simulink model "sim_Start_2021b"  (R2022a)
settings: Solver=FixedStepDiscrete  StartTime=0.0  StopTime=30  FixedStep=0.01  RelTol=1e-3
undefined symbols (not defined in the file): InputPWM, WheelSpeed
libraries: mobileRoboticsTrainingLib x6, simulink x2
settings Model: Creator=Boitumelo  LastModifiedBy=Admin
settings DebuggingCC: UnconnectedInputMsg=warning  UnconnectedOutputMsg=warning  UnconnectedLineMsg=warning
settings RTWCC: DLArmComputeVersion=19.05

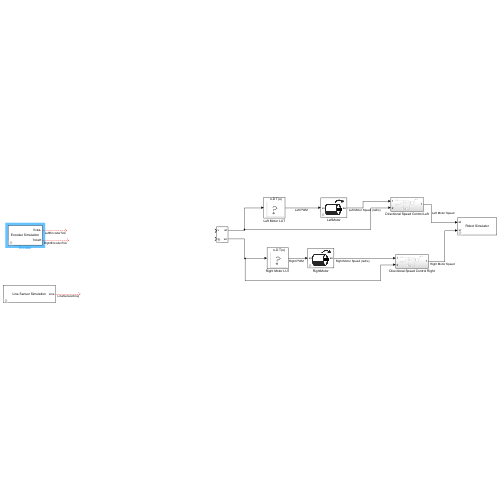
[thumbnail: Simulink's stored preview of the top-level diagram]
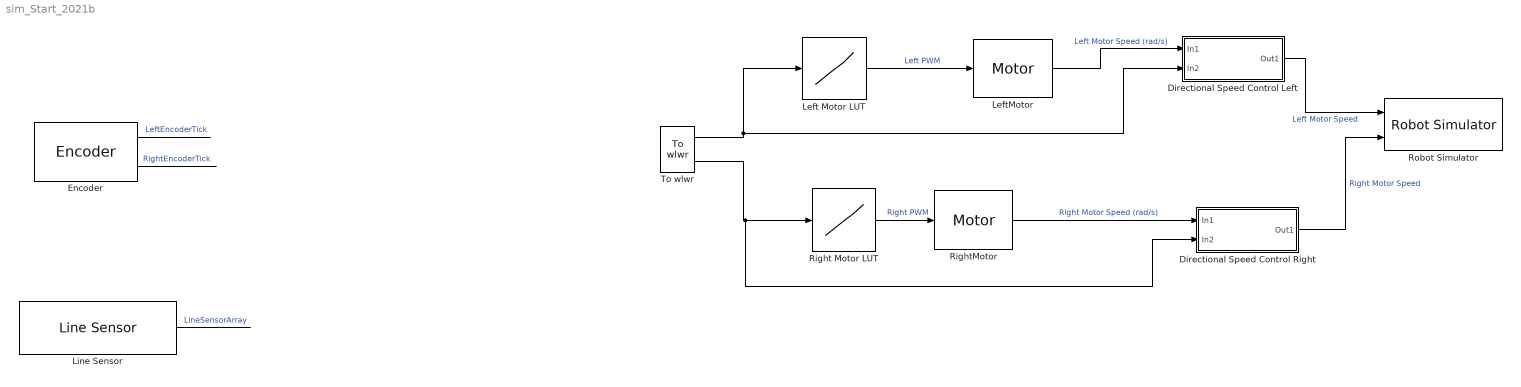
== system sim_Start_2021b ==
  Directional Speed Control Left : Subsystem
  Directional Speed Control Right : Subsystem
  Encoder : mobileRoboticsTrainingLib/Encoder  axleLength=axleLength  wheelR=wheelR  ticksPerRot=ticksPerRot
      settings: SourceProductName=Mobile Robotics Training Library
  Left Motor LUT : Lookup_n-D  NumberOfTableDimensions=1  BreakpointsForDimension1=WheelSpeed  Table=InputPWM  InterpMethod=Nearest  ExtrapMethod=Clip  InternalRulePriority=Speed  RndMeth=Simplest
  LeftMotor : mobileRoboticsTrainingLib/Motor  motorPlant=wheelMotorModel  sensorType=Speed
      settings: SourceProductName=Mobile Robotics Training Library
  Line Sensor : mobileRoboticsTrainingLib/Line Sensor  mapVariable=mapForSim  envVal=1  lineVal=0  sensOff=[0 0; 0 0; 0 0; 0 0]
      settings: SourceProductName=Mobile Robotics Training Library
  Right Motor LUT : Lookup_n-D  NumberOfTableDimensions=1  BreakpointsForDimension1=WheelSpeed  Table=InputPWM  InterpMethod=Nearest  ExtrapMethod=Clip  InternalRulePriority=Speed  RndMeth=Simplest
  RightMotor : mobileRoboticsTrainingLib/Motor  motorPlant=wheelMotorModel  sensorType=Speed
      settings: SourceProductName=Mobile Robotics Training Library
  Robot Simulator : mobileRoboticsTrainingLib/Robot Simulator  Priority=99  mapVar=mapForSim  startX=0.2126  startY=0.077048  startTheta=0  axleLength=axleLength  wheelR=wheelR
  To wlwr : mobileRoboticsTrainingLib/To wlwr  axleLength=0.1  wheelR=0.05
  wires:
  Directional Speed Control Left/1(Out1) -> Robot Simulator/1  "Left Motor Speed"
  Right Motor LUT/1 -> RightMotor/1  "Right PWM"
  Left Motor LUT/1 -> LeftMotor/1  "Left PWM"
  Encoder/1 -> ?  "LeftEncoderTick"
  Encoder/2 -> ?  "RightEncoderTick"
  To wlwr/1 -> Directional Speed Control Left/2(In2), Left Motor LUT/1
  To wlwr/2 -> Directional Speed Control Right/2(In2), Right Motor LUT/1
  Line Sensor/1 -> ?  "LineSensorArray"
  RightMotor/1 -> Directional Speed Control Right/1(In1)  "Right Motor Speed (rad/s)"
  LeftMotor/1 -> Directional Speed Control Left/1(In1)  "Left Motor Speed (rad/s)"
  Directional Speed Control Right/1(Out1) -> Robot Simulator/2  "Right Motor Speed"

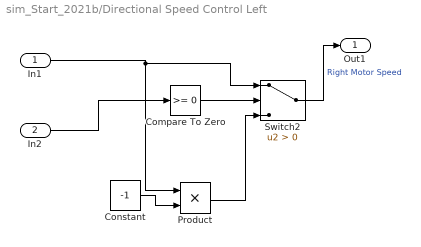
== system sim_Start_2021b/Directional Speed Control Left ==
  In1 : Inport
  In2 : Inport  Port=2
  Compare To Zero : simulink/Logic and Bit Operations/Compare To Zero  relop=>=  OutDataTypeStr=boolean
  Constant : Constant  Value=-1
  Product : Product
  Switch2 : Switch  Criteria=u2 > Threshold  SaturateOnIntegerOverflow=off  InputSameDT=off
  Out1 : Outport
  wires:
  Compare To Zero/1 -> Switch2/2
  In1/1 -> Switch2/1, Product/1
  Constant/1 -> Product/2
  Product/1 -> Switch2/3
  In2/1 -> Compare To Zero/1
  Switch2/1 -> Out1/1  "Right Motor Speed"

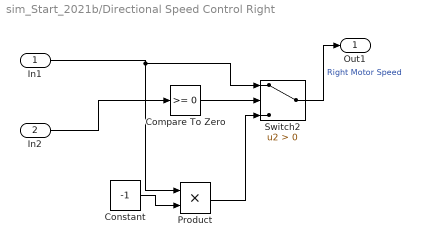
== system sim_Start_2021b/Directional Speed Control Right ==
  In1 : Inport
  In2 : Inport  Port=2
  Compare To Zero : simulink/Logic and Bit Operations/Compare To Zero  relop=>=  OutDataTypeStr=boolean
  Constant : Constant  Value=-1
  Product : Product
  Switch2 : Switch  Criteria=u2 > Threshold  SaturateOnIntegerOverflow=off  InputSameDT=off
  Out1 : Outport
  wires:
  Compare To Zero/1 -> Switch2/2
  In1/1 -> Switch2/1, Product/1
  Constant/1 -> Product/2
  Product/1 -> Switch2/3
  In2/1 -> Compare To Zero/1
  Switch2/1 -> Out1/1  "Right Motor Speed"
